simulink model "P4"  (R2021b)
settings: Solver=VariableStepAuto  StartTime=0.0  StopTime=100.0  RelTol=1e-3
libraries: fuzblock x1
settings Model: Creator=Pablo  LastModifiedBy=Pablo

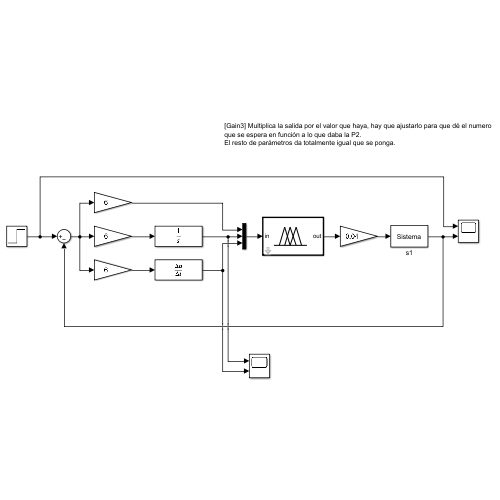
[thumbnail: Simulink's stored preview of the top-level diagram]
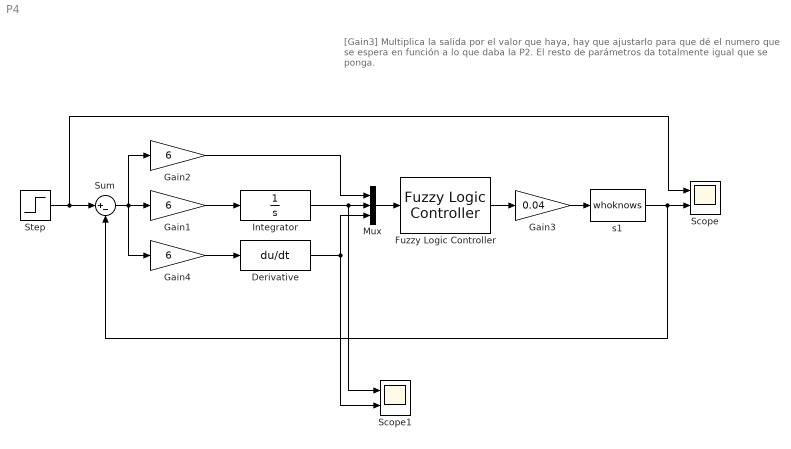
== system P4 ==
  note: [Gain3] Multiplica la salida por el valor que haya, hay que ajustarlo para que dé el numero que se espera en función a lo que daba la P2.
      | El resto de parámetros da totalmente igual que se ponga.
  Derivative : Derivative
  Fuzzy Logic Controller : fuzblock/Fuzzy Logic  Controller  FIS='Fuzzy3.fis'  OutputSampleNumber=101  DataType=double  FuzzifiedInputs=off  RuleFiringStrengths=off  RuleOutputs=off  AggregatedOutputs=off  SimulateUsing=Interpreted execution  OutOfRangeInputValueMessage=warning  NoRuleFiredMessage=warning  EmptyOutputFuzzySetMessage=warning
  Gain1 : Gain  Gain=6
  Gain2 : Gain  Gain=6
  Gain3 : Gain  Gain=0.04
  Gain4 : Gain  Gain=6
  Integrator : Integrator
  Mux : Mux  Inputs=3
  Scope : Scope  NumInputPorts=2
  Scope1 : Scope  NumInputPorts=2
  Step : Step  SampleTime=0
  Sum : Sum  Inputs=|+-
  s1 : M-S-Function  FunctionName=whoknows  Parameters=L, P1, P2, T, R  mask{L=4, P1=1, P2=1, T=2, R=0}
      mask prompts: L "Laboratorio"; P1 "Primer digito del Puesto"; P2 "Segundo digito del Puesto"; T "Tipo de Planta"; R "Ruido"
      mask Display: disp('Sistema')
  wires:
  s1/1 -> Sum/2, Scope/2
  Step/1 -> Scope/1, Sum/1
  Mux/1 -> Fuzzy Logic Controller/1
  Sum/1 -> Gain4/1, Gain2/1, Gain1/1
  Gain1/1 -> Integrator/1
  Integrator/1 -> Mux/2, Scope1/1
  Derivative/1 -> Mux/3, Scope1/2
  Gain3/1 -> s1/1
  Fuzzy Logic Controller/1 -> Gain3/1
  Gain2/1 -> Mux/1
  Gain4/1 -> Derivative/1
